simulink model "Events1"  (Simulink 5.0)
settings: Solver=ode45  StartTime=0.0  StopTime=10.0  RelTol=1e-3
settings Model: Creator=scaife  LastModifiedBy=scaife  ExtModeAutoUpdateStatusClock=off

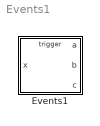
== system Events1 ==
  Events1 : Stateflow chart

== stateflow chart Events1 ==
  state A [parallel]
    state A2
      state A2a/
        en:a=x+3
      state A2b/
        en:a=x+4
      (default) -> A2a
      A2b -> A2a : R/R1
      A2a -> A2b : S/S1
    state A1
      state A1a/
        en:a=x+1
      state A1b/
        en:a=x+2
      (default) -> A1a
      A1a -> A1b : S/S1
      A1b -> A1a : R/R1
    (default) -> A1
    A1 -> A2 : T/T1
    A2 -> A1 : T/T1
  state B [parallel]
    state B2
      state B2a/
        en:b=x+7
      state B2b/
        en:b=x+8
      (default) -> B2a
      B2b -> B2a : R1
      B2a -> B2b : S1
    state B1
      state B1a/
        en:b=x+5
      state B1b/
        en:b=x+6
      (default) -> B1a
      B1b -> B1a : R1
      B1a -> B1b : S1
    (default) -> B1
    B1 -> B2 : T1/c++
    B2 -> B1 : T1/c++
  data: a output int32; x input int32; b output int32; c output int32
  events: R1 local EITHER_EDGE_EVENT; S1 local EITHER_EDGE_EVENT; T1 local EITHER_EDGE_EVENT; R input EITHER_EDGE_EVENT; S input EITHER_EDGE_EVENT; T input EITHER_EDGE_EVENT
